simulink model "mod2_errorfeedback"  (Simulink 8.1)
settings: Solver=FixedStepDiscrete  StartTime=0.0  StopTime=80e-3  RelTol=1e-3
undefined symbols (not defined in the file): Fs, modctrl
libraries: dspsigops x2, dspsrcs4 x1
settings Model: Creator=amyles  LastModifiedBy=amyles
settings DataIOCC: LimitDataPoints=off  MaxDataPoints=50000
settings OptimizationCC: InlineParams=on
settings DebuggingCC: StrictBusMsg=Warning
settings ModelReferenceCC: ModelReferenceNumInstancesAllowed=Single

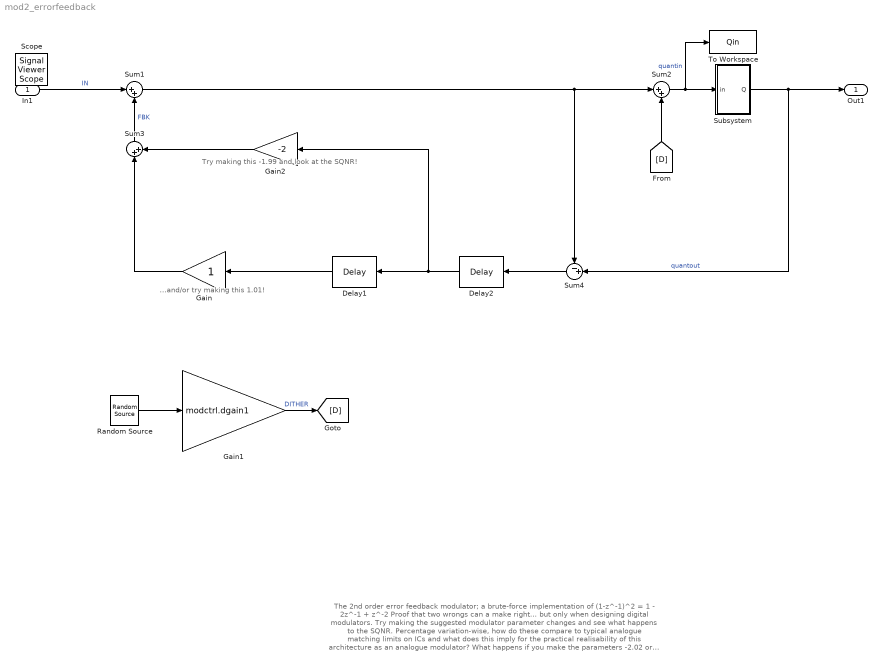
== system mod2_errorfeedback ==
  note: The 2nd order error feedback modulator; a brute-force implementation of (1-z^-1)^2 = 1 - 2z^-1 + z^-2
      |
      | Proof that two wrongs can a make right... but only when designing digital modulators. Try making
      | the suggested modulator parameter changes and see what happens to the SQNR. Percentage
      | variation-wise, how do these compare to typical analogue matching limits on ICs and what
      | does this imply for the practical realisability of this architecture as an analogue modulator?
      | What happens if you make the parameters -2.02 or 0.98? Why? Can you confirm this by SQNR
      | hand calculation (a good test that you understand what is going on and general modulator analysis)?
      | (Hint: Decompose  the NTF when there are coefficient errors into (1+z^-1)^2 + (other terms) and
      | then figure-out what (other terms) do to the noise in the signal band).
  note: ...and/or try making this 1.01!
  note: Try making this -1.99
      | and look at the SQNR!
  In1 : Inport
  Delay1 : dspsigops/Delay  InputProcessing=Inherited (this choice will be removed - see release notes)  dly_unit=Samples  delay=1  ic_detail=off  dif_ic_for_ch=off  dif_ic_for_dly=off  ic=0  reset_popup=None
  Delay2 : dspsigops/Delay  InputProcessing=Inherited (this choice will be removed - see release notes)  dly_unit=Samples  delay=1  ic_detail=off  dif_ic_for_ch=off  dif_ic_for_dly=off  ic=0  reset_popup=None
  Gain : Gain
  Gain1 : Gain  Gain=modctrl.dgain1
      settings: AttributesFormatString=Dither level adjust
  Gain2 : Gain  Gain=-2
  Random Source : dspsrcs4/Random Source  SrcType=Uniform  NormMethod=Ziggurat  CltLength=12  MinVal=-1  MaxVal=1  MeanVal=0  VarVal=1  RepMode=Not repeatable  rawSeed=1  IsInherit=off  SampMode=Discrete  SampTime=1/Fs  SampFrame=1  DataType=Double  OutComplex=Real
      settings: AttributesFormatString=Dither source
  Subsystem : Subsystem
      settings: AttributesFormatString=1-bit quantiser
  Sum1 : Sum  Inputs=|++
      settings: AttributesFormatString=Modulator input\nloop servo error (input - fbk)
  Sum2 : Sum  Inputs=|++
  Sum3 : Sum  Inputs=|++
  Sum4 : Sum  Inputs=-+|
  To Workspace : ToWorkspace  VariableName=Qin  SampleTime=-1  SaveFormat=Structure
  Out1 : Outport
  Scope : SignalViewerScope  IOType=viewer  ZoomMode=xonly  RefreshTime=0.035000
  wires:
  Delay2/1 -> Delay1/1, Gain2/1
  In1/1 -> Sum1/1  "IN"
  Sum2/1 -> Subsystem/1(in), To Workspace/1  "quantin"
  Subsystem/1(Q) -> Out1/1, Sum4/2  "quantout"
  Random Source/1 -> Gain1/1
  Delay1/1 -> Gain/1
  Gain/1 -> Sum3/1
  Sum3/1 -> Sum1/2  "FBK"
  Gain2/1 -> Sum3/2
  Sum4/1 -> Delay2/1
  Sum1/1 -> Sum2/1, Sum4/1
  Gain1/1 -> [D]  "DITHER"
  [D] -> Sum2/2

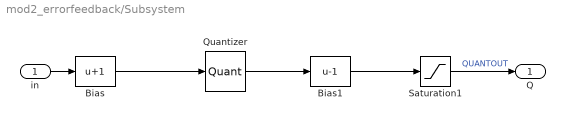
== system mod2_errorfeedback/Subsystem ==
  in : Inport
  Bias : Bias  Bias=1
      settings: AttributesFormatString=Need offset to give\nMID-RISE quantiser
  Bias1 : Bias  Bias=-1
  Quantizer : Quantizer  QuantizationInterval=2  LinearizeAsGain=off
  Saturation1 : Saturate  UpperLimit=1  LowerLimit=-1
      settings: AttributesFormatString=Limit quantiser\noutput to +/-1
  Q : Outport
  wires:
  Bias/1 -> Quantizer/1
  Quantizer/1 -> Bias1/1
  Bias1/1 -> Saturation1/1
  in/1 -> Bias/1
  Saturation1/1 -> Q/1  "QUANTOUT"
